simulink model "Drone"  (R2022b)
settings: Solver=ode4  StartTime=0.0  StopTime=20  FixedStep=1e-3  RelTol=1e-3
PreLoadFcn:
  | Parametri_Drone
values from neighbouring files (symbols this model uses):
  aeta0 = [ab0 0 0 ... (first row only)    [Parametri_Drone.m]    (also in Parametri_Drone.mat = [150  0  0; 0  150  0; 0  0  12])
  aeta1 = [ab1 0 0 ... (first row only)    [Parametri_Drone.m]    (also in Parametri_Drone.mat = [35  0  0; 0  35  0; 0  0  7])
  ax0 = x(3)    [Parametri_Drone.m]    (also in Parametri_Drone.mat = 2.25)
  ax1 = x(2)    [Parametri_Drone.m]    (also in Parametri_Drone.mat = 3)
  ay0 = y(3)    [Parametri_Drone.m]    (also in Parametri_Drone.mat = 2.25)
  ay1 = y(2)    [Parametri_Drone.m]    (also in Parametri_Drone.mat = 3)
  az0 = a(3)    [Parametri_Drone.m]    (also in Parametri_Drone.mat = 9)
  az1 = a(2)    [Parametri_Drone.m]    (also in Parametri_Drone.mat = 6)
  e3T = e3'    [Parametri_Drone.m]    (also in Parametri_Drone.mat = [0 0 1])
  F = [  1          1           1           1 ... (first row only)    [Parametri_Drone.m]    (also in Parametri_Drone.mat = [1 0 -0.45 -0.0239616613419 1 0.45 0 0.0239616613419 1 0 0.4)
  F1 = [0 0 0 0 ... (first row only)    [Parametri_Drone.m]    (also in Parametri_Drone.mat = [0  0  0  0; 0  0  0  0; 1  1  1  1]; Parametri_Drone1.m)
  F2 = [ 0         l          0         -l ... (first row only)    [Parametri_Drone.m]    (also in Parametri_Drone.mat = [0  0.45  0  -0.45; -0.45  0  0.45  0; -0.0239616613419  0.0; Parametri_Drone1.m)
  g = 9.81    [Parametri_Drone.m]    (also in Parametri_Drone.mat; Parametri_Drone1.m)
  J = [J_x  0    0 ... (first row only)    [Parametri_Drone.m]    (also in Parametri_Drone.mat = [0.363  0  0; 0  0.363  0; 0  0  0.651]; Parametri_Drone1.m)
  K_r = 0    [Parametri_Drone.m]    (also in Parametri_Drone.mat; Parametri_Drone1.m)
  K_t = 0    [Parametri_Drone.m]    (also in Parametri_Drone.mat; Parametri_Drone1.m)
  L1 = [l0 0 0 ... (first row only)    [Parametri_Drone.m]    (also in Parametri_Drone.mat = [6  0  0; 0  11  0; 0  0  6])
  L2 = [l_0 0 0 ... (first row only)    [Parametri_Drone.m]    (also in Parametri_Drone.mat = [6  0  0; 0  11  0; 0  0  6])
  m = 3.95    [Parametri_Drone.m]    (also in Parametri_Drone.mat; Parametri_Drone1.m)
settings Model: Creator=eris4  LastModifiedBy=Denil
settings ModelReferenceCC: EnableRefExpFcnMdlSchedulingChecks=on

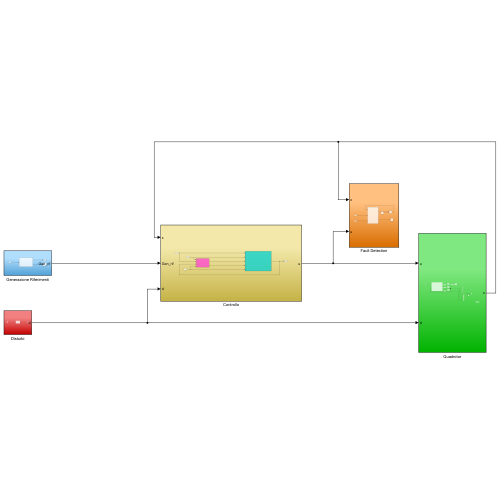
[thumbnail: Simulink's stored preview of the top-level diagram]
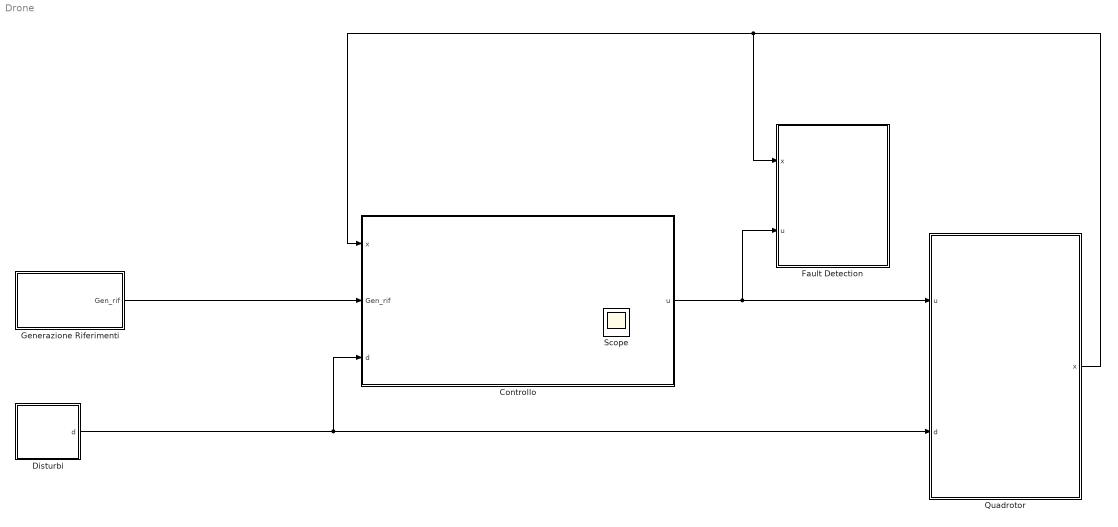
== system Drone ==
  Controllo : Subsystem
  Disturbi : Subsystem
  Fault Detection : Subsystem
  Generazione Riferimenti : Subsystem
  Quadrotor : Subsystem
  Scope : Scope
  wires:
  Generazione Riferimenti/1(Gen_rif) -> Controllo/2(Gen_rif)
  Controllo/1(u) -> Fault Detection/2(u), Quadrotor/1(u)
  Quadrotor/1(x) -> Controllo/1(x), Fault Detection/1(x)
  Disturbi/1(d) -> Controllo/3(d), Quadrotor/2(d)

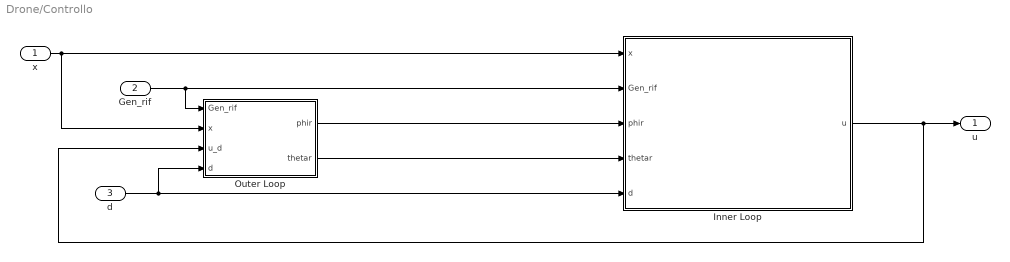
== system Drone/Controllo ==
  x : Inport
  Gen_rif : Inport  Port=2
  d : Inport  Port=3
  Inner Loop : Subsystem
  Outer Loop : Subsystem
  u : Outport
  wires:
  Inner Loop/1(u) -> Outer Loop/3(u_d), u/1
  x/1 -> Inner Loop/1(x), Outer Loop/2(x)
  Gen_rif/1 -> Outer Loop/1(Gen_rif), Inner Loop/2(Gen_rif)
  Outer Loop/1(phir) -> Inner Loop/3(phir)
  Outer Loop/2(thetar) -> Inner Loop/4(thetar)
  d/1 -> Inner Loop/5(d), Outer Loop/4(d)

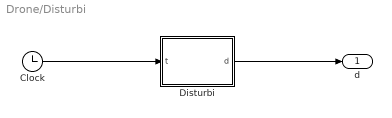
== system Drone/Disturbi ==
  Clock : Clock
  Disturbi : MATLAB Function  TreatAsAtomicUnit=on
  d : Outport
  wires:
  Disturbi/1(d) -> d/1
  Clock/1 -> Disturbi/1(t)

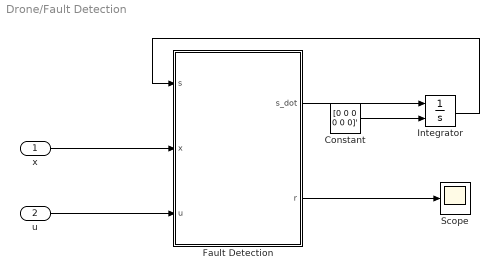
== system Drone/Fault Detection ==
  x : Inport
  u : Inport  Port=2
  Constant : Constant  Value=[0 0 0 0 0 0]'  VectorParams1D=off
  Fault Detection : MATLAB Function  TreatAsAtomicUnit=on
  Integrator : Integrator  InitialConditionSource=external
  Scope : Scope
  wires:
  x/1 -> Fault Detection/2(x)
  Fault Detection/1(s_dot) -> Integrator/1
  Integrator/1 -> Fault Detection/1(s)
  Fault Detection/2(r) -> Scope/1
  u/1 -> Fault Detection/3(u)
  Constant/1 -> Integrator/2

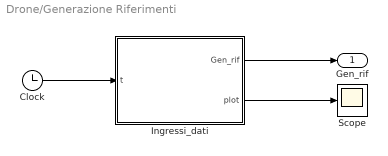
== system Drone/Generazione Riferimenti ==
  Clock : Clock
  Ingressi_dati : MATLAB Function  TreatAsAtomicUnit=on
  Scope : Scope
  Gen_rif : Outport
  wires:
  Clock/1 -> Ingressi_dati/1(t)
  Ingressi_dati/1(Gen_rif) -> Gen_rif/1
  Ingressi_dati/2(plot) -> Scope/1

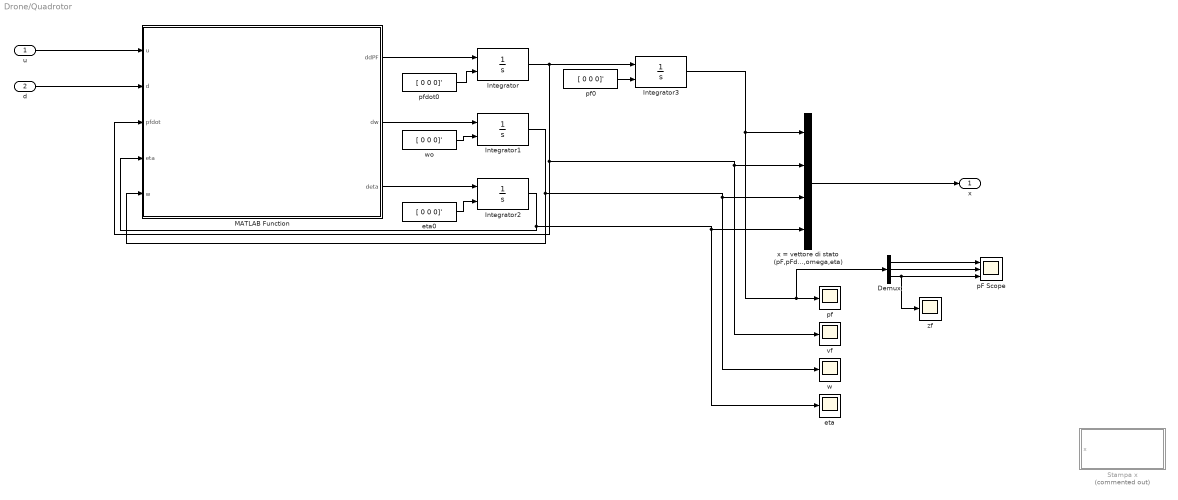
== system Drone/Quadrotor ==
  u : Inport
  d : Inport  Port=2
  Demux : Demux  Outputs=3
  Integrator{,1..3} (4 alike) : Integrator  InitialConditionSource=external
  MATLAB Function : MATLAB Function  TreatAsAtomicUnit=on
  Stampa x : MATLAB Function  Commented=on  TreatAsAtomicUnit=on
  eta : Scope
  eta0 : Constant  Value=[ 0 0 0]'
  pF Scope : Scope  NumInputPorts=3
  pf : Scope
  pf0 : Constant  Value=[ 0 0 0]'
  pfdot0 : Constant  Value=[ 0 0 0]'
  vf : Scope
  w : Scope
  wo : Constant  Value=[ 0 0 0]'
  x = vettore di stato (pF,pFdot,omega,eta) : Mux
  zf : Scope
  x : Outport
  wires:
  Integrator1/1 -> MATLAB Function/5(w), w/1, x = vettore di stato (pF,pFdot,omega,eta)/3
  Integrator2/1 -> MATLAB Function/4(eta), eta/1, x = vettore di stato (pF,pFdot,omega,eta)/4
  Integrator/1 -> Integrator3/1, x = vettore di stato (pF,pFdot,omega,eta)/2, vf/1, MATLAB Function/3(pfdot)
  x = vettore di stato (pF,pFdot,omega,eta)/1 -> x/1
  d/1 -> MATLAB Function/2(d)
  u/1 -> MATLAB Function/1(u)
  pfdot0/1 -> Integrator/2
  wo/1 -> Integrator1/2
  eta0/1 -> Integrator2/2
  MATLAB Function/2(dw) -> Integrator1/1
  MATLAB Function/1(ddPF) -> Integrator/1
  MATLAB Function/3(deta) -> Integrator2/1
  pf0/1 -> Integrator3/2
  Integrator3/1 -> x = vettore di stato (pF,pFdot,omega,eta)/1, Demux/1, pf/1
  Demux/3 -> zf/1, pF Scope/3
  Demux/2 -> pF Scope/2
  Demux/1 -> pF Scope/1

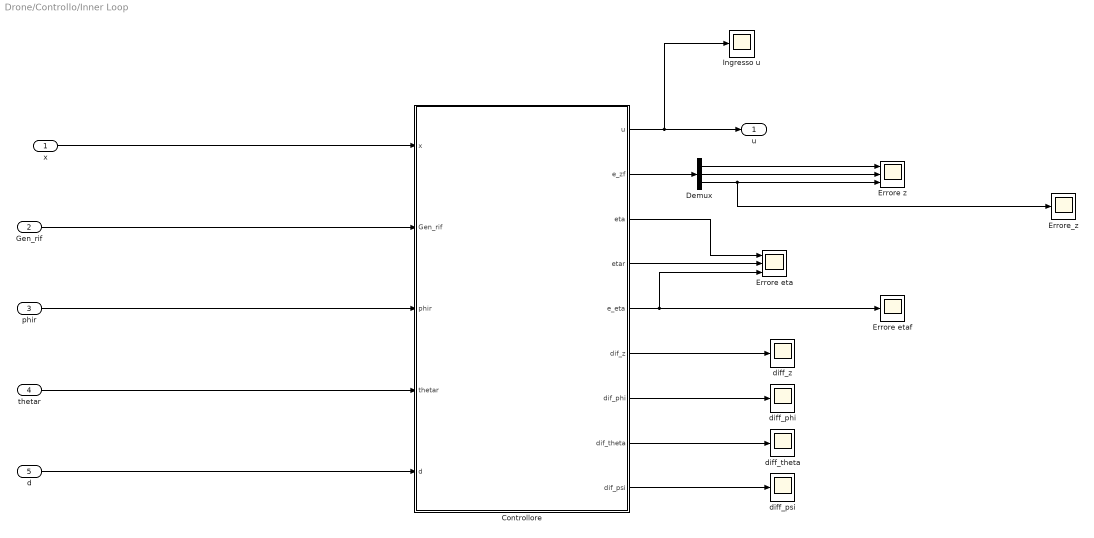
== system Drone/Controllo/Inner Loop ==
  x : Inport
  Gen_rif : Inport  Port=2
  phir : Inport  Port=3
  thetar : Inport  Port=4
  d : Inport  Port=5
  Controllore : MATLAB Function  TreatAsAtomicUnit=on
  Demux : Demux  Outputs=3
  Errore eta : Scope  NumInputPorts=3
  Errore etaf : Scope
  Errore z : Scope  NumInputPorts=3
  Errore_z : Scope
  Ingresso u : Scope
  diff_phi : Scope
  diff_psi : Scope
  diff_theta : Scope
  diff_z : Scope
  u : Outport
  wires:
  Controllore/1(u) -> u/1, Ingresso u/1
  Gen_rif/1 -> Controllore/2(Gen_rif)
  x/1 -> Controllore/1(x)
  d/1 -> Controllore/5(d)
  Controllore/2(e_zf) -> Demux/1
  Demux/1 -> Errore z/1
  Demux/3 -> Errore_z/1, Errore z/3
  Demux/2 -> Errore z/2
  Controllore/3(eta) -> Errore eta/1
  Controllore/4(etar) -> Errore eta/2
  Controllore/5(e_eta) -> Errore eta/3, Errore etaf/1
  Controllore/6(dif_z) -> diff_z/1
  Controllore/7(dif_phi) -> diff_phi/1
  Controllore/8(dif_theta) -> diff_theta/1
  Controllore/9(dif_psi) -> diff_psi/1
  phir/1 -> Controllore/3(phir)
  thetar/1 -> Controllore/4(thetar)

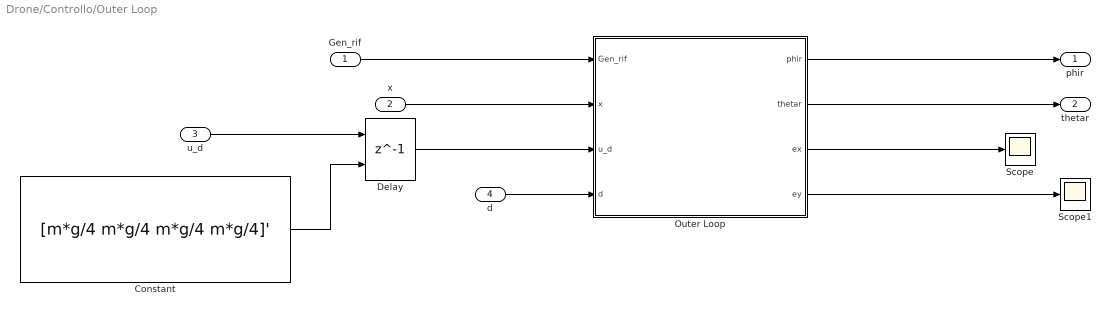
== system Drone/Controllo/Outer Loop ==
  Gen_rif : Inport
  x : Inport  Port=2
  u_d : Inport  Port=3
  d : Inport  Port=4
  Constant : Constant  Value=[m*g/4 m*g/4 m*g/4 m*g/4]'  VectorParams1D=off
  Delay : Delay  DelayLength=1  InitialConditionSource=Input port  InitialCondition=1
      settings: InputPortMap=u0,p4
  Outer Loop : MATLAB Function  TreatAsAtomicUnit=on
  Scope : Scope
  Scope1 : Scope
  phir : Outport
  thetar : Outport  Port=2
  wires:
  Constant/1 -> Delay/2
  Delay/1 -> Outer Loop/3(u_d)
  d/1 -> Outer Loop/4(d)
  u_d/1 -> Delay/1
  Outer Loop/2(thetar) -> thetar/1
  Outer Loop/1(phir) -> phir/1
  Gen_rif/1 -> Outer Loop/1(Gen_rif)
  x/1 -> Outer Loop/2(x)
  Outer Loop/3(ex) -> Scope/1
  Outer Loop/4(ey) -> Scope1/1

== matlab function Drone/Disturbi/Disturbi ==
  data: d output; t input
function d = Disturbi(t)
if t<=10
%deltam

    deltamx=0;
    deltamy=0;
    deltamz=0;


    %deltaf
    deltafx=0;
    deltafy=0;
    deltafz=0;


    %fe
    fex=0;
    fey=0;
    fez=0;
elseif t>15
    deltamx= 16/5;
    deltamy= 16/5;
    deltamz= 16/5;
    deltafx= 16/5;
    deltafy= 16/5;
    deltafz= 16/5;
    fex= 16/5;
    fey= 16/5;
    fez= 16/5;
else

    deltamx= (t+sin(t))/5;
    deltamy= (t+sin(t))/5;
    deltamz= (t+sin(t))/5;
    deltafx= (t+sin(t))/5;
    deltafy= (t+sin(t))/5;
    deltafz= (t+sin(t))/5;
    fex= (t+sin(t))/5;
    fey= (t+sin(t))/5;
    fez= (t+sin(t))/5;

   
end
d=[deltamx deltamy deltamz deltafx deltafy deltafz fex fey fez]';

== matlab function Drone/Controllo/Outer Loop/Outer Loop ==
  data: Gen_rif input; phir output; x input; u_d input; d input; m parameter; K_t parameter; thetar output; ax0 parameter; ay0 parameter; ax1 parameter; ay1 parameter; ex output; ey output
function [phir,thetar,ex,ey] = Outerloop(Gen_rif,x,u_d,d,m, K_t,ax0, ay0, ax1, ay1)
%pf
xf=x(1);
yf=x(2);

%pfdot
pFdot = x(4:6);
xFdot=pFdot(1);
yFdot=pFdot(2);
%fe
Fe=d(7:9);
Fex=Fe(1);
Fey=Fe(2);

%Delta_F_m_B

deltaF_m_B=d(4:6);
delta_f_z=deltaF_m_B(3);

% fz
fz=[1 1 1 1]*u_d;

% Angoli
eta = x(10:12);
psi = eta(3);

matr=[sin(psi) cos(psi);
      -cos(psi) sin(psi)];
%errori
xfr=Gen_rif(1);
yfr=Gen_rif(2);

dxfr=Gen_rif(4);
dyfr=Gen_rif(5);
ddxfr=Gen_rif(7);
ddyfr=Gen_rif(8);

vx=ddxfr -ax1*(xFdot- dxfr) - ax0*(xf-xfr);
vy=ddyfr -ay1*(yFdot- dyfr) - ay0*(yf-yfr);

ex=xf-xfr;
ey=yf-yfr;

y=(m/(fz + delta_f_z))*(inv(matr)*((K_t/m)*[xFdot yFdot]' -(1/m)*[Fex Fey]' +[vx vy]'));
phir=y(1);
thetar=y(2);

== matlab function Drone/Fault Detection/Fault Detection ==
  data: s input; x input; s_dot output; r output; u input; F1 parameter; J parameter; m parameter; F2 parameter; K_t parameter; K_r parameter; e3 parameter; g parameter; L1 parameter; L2 parameter
function [s_dot, r] = Fault_Detection(s, x, u,F1, J, m, F2, K_t, K_r, e3, g,L1, L2)
pfdot = x(4:6);
pfdot1=pfdot(1);
pfdot2=pfdot(2);
pfdot3=pfdot(3);
z1=s(1:3);
z11=z1(1);
z12=z1(2);
z13=z1(3);

z2=s(4:6);
z21=z2(1);
z22=z2(2);
z23=z2(3);
eta = x(10:12);
phi= eta(1);
theta = eta(2);
psi = eta(3);
w=x(7:9);
wd1=w(1);
wd2=w(2);
wd3=w(3);
%w_d=[wd1 wd2 wd3]';

R =[cos(psi)*cos(theta) cos(psi)*sin(phi)*sin(theta)-cos(phi)*sin(psi) sin(phi)*sin(psi)+cos(phi)*cos(psi)*sin(theta);
    cos(theta)*sin(psi) cos(phi)*cos(psi)+sin(phi)*sin(psi)*sin(theta) cos(phi)*sin(psi)*sin(theta)-cos(psi)*sin(phi);
    -sin(theta)         cos(theta)*sin(phi)                            cos(phi)*cos(theta)];

Fm= F1*u;
Mm=F2*u;

ddPF=(-K_t*pfdot -m*g*e3 +R*Fm +L1*(pfdot-z1) )/m ;
dw= inv(J)*(-K_r*w -cross(w,(J*w)) + Mm) +L2*(w-z2);

xddpf=ddPF(1);
yddpf=ddPF(2);
zddpf=ddPF(3);

xdw=dw(1);
ydw=dw(2);
zdw=dw(3);
s_dot=[xddpf yddpf zddpf xdw ydw zdw]';
x_d=[pfdot1 pfdot2 pfdot3 wd1 wd2 wd3]';

z=[z11 z12 z13 z21 z22 z23]';

r=norm(x_d - z)

== matlab function Drone/Controllo/Inner Loop/Controllore ==
  data: x input; Gen_rif input; phir input; thetar input; d input; u output; F parameter; e3T parameter; J parameter; e3 parameter; g parameter; m parameter; K_t parameter; K_r parameter; aeta0 parameter; aeta1 parameter; az1 parameter; az0 parameter; e_zf output; eta output; etar output; e_eta output; dif_z output; dif_phi output; dif_theta output; dif_psi output
function [u,e_zf,eta,etar,e_eta,dif_z,dif_phi,dif_theta,dif_psi] =Controllo(x,Gen_rif,phir,thetar,d,F,e3T,J,e3, g, m, K_t, K_r,aeta0, aeta1, az1, az0)

u = [0 0 0 0]';

%% Unzip vettore di stato
pF = x(1:3);
pFdot = x(4:6);
w = x(7:9);
eta = x(10:12);

phi= eta(1);
theta = eta(2);
psi = eta(3);

psir=Gen_rif(10);
etar=[phir thetar psir]';

p=w(1);
q=w(2);
r=w(3);


zf = pF(3);
dzf = pFdot(3);

zfr=Gen_rif(3);

deltam=d(1:3);
fe=d(7:9);
%% Matrice R

R =[cos(psi)*cos(theta) cos(psi)*sin(phi)*sin(theta)-cos(phi)*sin(psi) sin(phi)*sin(psi)+cos(phi)*cos(psi)*sin(theta);
    cos(theta)*sin(psi) cos(phi)*cos(psi)+sin(phi)*sin(psi)*sin(theta) cos(phi)*sin(psi)*sin(theta)-cos(psi)*sin(phi);
    -sin(theta)         cos(theta)*sin(phi)                            cos(phi)*cos(theta)];

%% Matrice T

T=[1 sin(phi)*tan(theta) cos(phi)*tan(theta);
   0 cos(phi)            -sin(phi);
   0 sin(phi)/cos(theta) cos(phi)/cos(theta)];

%% Derivata Matrice T

d_T= [0          cos(phi)*tan(theta)*(p + r*cos(phi)*tan(theta) + q*sin(phi)*tan(theta)) + sin(phi)*(tan(theta)^2 + 1)*(q*cos(phi) - r*sin(phi))          cos(phi)*(tan(theta)^2 + 1)*(q*cos(phi) - r*sin(phi)) - sin(phi)*tan(theta)*(p + r*cos(phi)*tan(theta) + q*sin(phi)*tan(theta));
      0                                                                            -sin(phi)*(p + r*cos(phi)*tan(theta) + q*sin(phi)*tan(theta))                                                                            -cos(phi)*(p + r*cos(phi)*tan(theta) + q*sin(phi)*tan(theta));
      0 (cos(phi)*(p + r*cos(phi)*tan(theta) + q*sin(phi)*tan(theta)))/cos(theta) + (sin(phi)*sin(theta)*(q*cos(phi) - r*sin(phi)))/cos(theta)^2 (cos(phi)*sin(theta)*(q*cos(phi) - r*sin(phi)))/cos(theta)^2 - (sin(phi)*(p + r*cos(phi)*tan(theta) + q*sin(phi)*tan(theta)))/cos(theta)];
 

%% r33
 
r33=e3T*R*e3;

%% Inversa di A

A = [(1/m)*r33 zeros(1,3); 
    zeros(3,1) T*inv(J)];
Ainv = inv(A);

%% Calcolo di bz

bz=-K_t/m*dzf -g +1/m*e3T*fe;

%% Calcolo di beta

beta= d_T*w -K_t*T*inv(J)*w -T*inv(J)*(cross(w,J*w)) +T*inv(J)*deltam;

%% Calcolo vz
dzfr = Gen_rif(6);
ddzfr= Gen_rif(9);

vz=ddzfr -az1*(dzf- dzfr) - az0*(zf-zfr);

%% Calcolo veta
dphir= Gen_rif(11);
dthetar= Gen_rif(12);
dpsir= Gen_rif(13);
detar = [dphir dthetar dpsir]';
ddphir= Gen_rif(14);
ddthetar= Gen_rif(15);
ddpsir= Gen_rif(16);
ddetar= [ddphir ddthetar ddpsir]';
veta=ddetar -aeta1*(T*w -detar) -aeta0*(eta-etar);

%% Calcolo dell'ingresso
u= inv(F)*Ainv*([-bz; -beta] + [vz; veta]);

%% Errore
e_z=(zfr-zf);
e_zf=[zf zfr e_z]';

e_eta=(etar-eta);
dif_z=[zf zfr]';
dif_phi=[phi phir]';
dif_theta=[theta thetar]';
dif_psi=[psi psir]';

== matlab function Drone/Quadrotor/MATLAB Function ==
  data: u input; ddPF output; d input; dw output; deta output; pfdot input; eta input; w input; F1 parameter; J parameter; m parameter; g parameter; F2 parameter; K_t parameter; K_r parameter; e3 parameter
function [ddPF, dw, deta] = Drone(u,d,pfdot, eta, w, F1,J, m, g, F2, K_t, K_r,e3 )
%% 
   % Forze Esterne
   deltaM_m_B=d(1:3);
   deltaF_m_B=d(4:6);
   Fe=d(7:9);
   % Angoli
   phi=eta(1);
   theta=eta(2);
   psi=eta(3);

   R =[cos(psi)*cos(theta) cos(psi)*sin(phi)*sin(theta)-cos(phi)*sin(psi) sin(phi)*sin(psi)+cos(phi)*cos(psi)*sin(theta);
    cos(theta)*sin(psi) cos(phi)*cos(psi)+sin(phi)*sin(psi)*sin(theta) cos(phi)*sin(psi)*sin(theta)-cos(psi)*sin(phi);
    -sin(theta)         cos(theta)*sin(phi)                            cos(phi)*cos(theta)];

   T=[1 sin(phi)*tan(theta) cos(phi)*tan(theta);
   0 cos(phi)            -sin(phi);
   0 sin(phi)/cos(theta) cos(phi)/cos(theta)];

   Fm= F1*u;
   Mm=F2*u;
   
   ddPF=(-K_t*pfdot -m*g*e3 +R*(Fm +deltaF_m_B) + Fe)/m;
   dw= inv(J)*(-K_r*w -cross(w,(J*w)) + Mm + deltaM_m_B);
   deta= T*w;

== matlab function Drone/Quadrotor/Stampa x ==
  data: x input
function Stampa(x)

x;

end

== matlab function Drone/Generazione Riferimenti/Ingressi_dati ==
  data: t input; Gen_rif output; plot output
function [Gen_rif, plot] =Ingresso(t)
i=3;
r=2;
w=2*pi/10;
% Tutti i riferimenti a zero(hoovering);
if i==0
   xr=0;
   yr=0;
   zr=0;
   psir=0;
   dxfr=0;
   ddxfr=0;
   dyfr=0;
   ddyfr=0;
   dzfr = 0;
   ddzfr=0;
   dpsir=0;
   ddpsir=0;
%Valori costanti
elseif i==1
   xr=1.5;
   yr=1;
   zr=1.7;
   psir=deg2rad(15);
   dxfr=0;
   ddxfr=0;
   dyfr =0;
   ddyfr=0;
   dzfr=0;
   ddzfr=0;
   dpsir=0;
   ddpsir=0;
% Circonferenza nel piano x-y, mentre z,psi costanti a zero
elseif i==2
   xr=r*cos(w*t);
   yr=r*sin(w*t);
   zr=0;
   psir=0;
   dxfr = -r*w*sin(w*t) ;
   ddxfr= -r*w^2*cos(w*t);
   dyfr = r*w*cos(w*t);
   ddyfr= -r*w^2*sin(w*t);
   dzfr = 0;
   ddzfr= 0;
   dpsir=0;
   ddpsir=0;
% Circonferenza nel piano x-y, rampa su z, psi costante (i.e. elica ascendente, senza yaw)
elseif i==3
    %w=, definire raggio e w 
   xr=r*cos(w*t);
   yr=r*sin(w*t);
   zr=t;
   psir=deg2rad(15);
   dxfr = -r*w*sin(w*t) ;
   ddxfr= -r*w^2*cos(w*t);
   dyfr = r*w*cos(w*t);
   ddyfr= -r*w^2*sin(w*t);
   dzfr = 1;
   ddzfr=0;
   dpsir=0;
   ddpsir=0;


end

dphir=0;
ddphir=0;
dthetar=0;
ddthetar=0;

Gen_rif=[xr yr zr dxfr dyfr dzfr ddxfr ddyfr ddzfr psir dphir dthetar dpsir ddphir ddthetar ddpsir]';
plot=[xr yr zr]';
